simulink model "untitled1"  (R2023b)
settings: Solver=VariableStepAuto  StartTime=0.0  StopTime=inf  RelTol=1e-3
libraries: ros2lib x1
settings Model: Creator=basten  LastModifiedBy=gilang

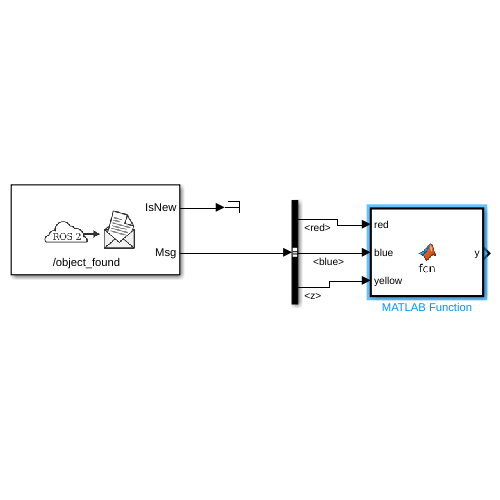
[thumbnail: Simulink's stored preview of the top-level diagram]
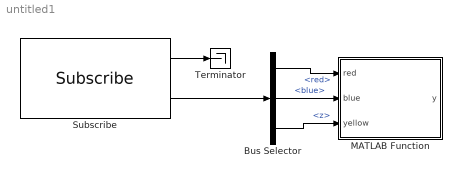
== system untitled1 ==
  Bus Selector : BusSelector  OutputSignals=red,blue,z
  MATLAB Function : MATLAB Function  TreatAsAtomicUnit=on
  Subscribe : ros2lib/Subscribe  topicSource=Select from ROS network  topic=/object_found  messageType=geometry_msgs/Point  sampleTime=0.01  QOSHistory=Keep last  QOSDepth=1  QOSReliability=Reliable  QOSDurability=Volatile
  Terminator : Terminator
  wires:
  Subscribe/2 -> Bus Selector/1
  Subscribe/1 -> Terminator/1
  Bus Selector/1 -> MATLAB Function/1(red)  "<red>"
  Bus Selector/2 -> MATLAB Function/2(blue)  "<blue>"
  Bus Selector/3 -> MATLAB Function/3(yellow)  "<z>"

== matlab function untitled1/MATLAB Function ==
  data: red input; y output; blue input; yellow input
function y = fcn(red, blue, yellow)

y = red;
